simulink model "test_engine"  (R2020a)
settings: Solver=VariableStepAuto  StartTime=0.0  StopTime=1.0  RelTol=1e-3
settings Model: Creator=malte  LastModifiedBy=malte

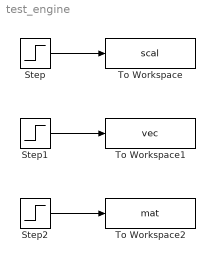
== system test_engine ==
  Step : Step  Before=1.2  After=3.4  SampleTime=0
  Step1 : Step  Before=[1.2, 3.4]  After=[5.6, 7.8]  SampleTime=0
  Step2 : Step  Before=[[1.2, 3.4, 5.6]; [7.8, 9.0, 1.2]]  After=[[3.4, 5.6, 7.8]; [9.0, 1.2, 3.4]]  SampleTime=0
  To Workspace : ToWorkspace  VariableName=scal  SaveFormat=Timeseries  SampleTime=1
  To Workspace1 : ToWorkspace  VariableName=vec  SaveFormat=Timeseries  SampleTime=1
  To Workspace2 : ToWorkspace  VariableName=mat  SaveFormat=Timeseries  SampleTime=1
  wires:
  Step1/1 -> To Workspace1/1
  Step/1 -> To Workspace/1
  Step2/1 -> To Workspace2/1
